simulink model "Arm11d"  (R2014b)
settings: Solver=ode23  StartTime=0.0  StopTime=4  MaxStep=0.005  RelTol=1e-3
values from neighbouring files (symbols this model uses):
  ArmIP = [2      0       -5;     -2      0       -5;           0      2       0;      0       -2      0;           -1     1       -6;     -1      -1      -6;           -1     1       -5;     -1      -1      -5;           0      -1.5    -6;      0      1.5     -15]    [params11c.m]    (also in params11cd.m; params11d.m)
  c = 1.12    [params11c.m]    (also in params11cd.m; params11d.m)
  d = 0.025    [params11c.m]    (also in params11cd.m; params11d.m)
  f1 = 0.82    [params11c.m]    (also in params11cd.m; params11d.m; piece5.m = sum(ar.*ar))
  f2 = 0.5    [params11c.m]    (also in params11cd.m; params11d.m; piece5.m = sum(cr.*cr))
  f3 = 0.43    [params11c.m]    (also in params11cd.m; params11d.m; piece5.m = sum(ar.*b))
  f4 = 0.58    [params11c.m]    (also in params11cd.m; params11d.m; piece5.m = sum(cr.*b))
  FarmIP = [0     1.5     -Larm-5;      0       -0.5    -Larm+3;            -1    1.5     -Larm-4]    [params11c.m]    (also in params11cd.m; params11d.m)
  Iarm = Iarm*10^(-4)    [params11c.m]    (also in params11cd.m; params11d.m)
  Ifarm = Ifarm*10^(-4)    [params11c.m]    (also in params11cd.m; params11d.m)
  kP = 2.58    [params11c.m]    (also in params11cd.m; params11d.m)
  Larm = 30    [params11c.m]    (also in params11cd.m; params11d.m)
  Lfarm = 26    [params11c.m]    (also in params11cd.m; params11d.m)
  Marm = dens*pi*(Rarm^2)*Larm    (= 2.35619449019)    [params11c.m]    (also in params11cd.m; params11d.m)
  Mfarm = dens*pi*(Rfarm^2)*Lfarm    (= 1.30690254389)    [params11c.m]    (also in params11cd.m; params11d.m)
  mu = 0.06    [params11c.m]    (also in params11cd.m; params11d.m)
  rhoP = 14.9    [params11c.m]    (also in params11cd.m; params11d.m)
  rlen = [13.8992; 12.5757; 9.1104; 7.1414; 17.4868; 17.7487; 18.8370;          17.8958; 33.5286; 22.2536; 16.9666]    [params11c.m]    (also in params11cd.m; params11d.m)
  tau = 0.01    [params11c.m]    (also in params11cd.m; params11d.m)
  tausq = tau^2    (= 0.0001)    [params11c.m]    (also in params11cd.m; params11d.m)
  vd = 0.15    [params11c.m]    (also in params11cd.m; params11d.m)
undefined symbols (not defined in the file or in its folder): geometry5, shaper2
libraries: mblibv1 x47, simulink x1
settings Model: Creator=sverduzco  LastModifiedBy=sergio
settings DataIOCC: SignalLoggingSaveFormat=ModelDataLogs
settings OptimizationCC: ExpressionDepthLimit=2147483647
settings DebuggingCC: UnderspecifiedInitializationDetection=Classic  MergeDetectMultiDrivingBlocksExec=none  FcnCallInpInsideContextMsg=UseLocalSettings  StateNameClashWarn=warning
settings GRTTargetCC: CombineOutputUpdateFcns=off  GRTInterface=on
settings SimMechanicsCC: VisOnUpdateDiagram=on  VisDuringSimulation=on

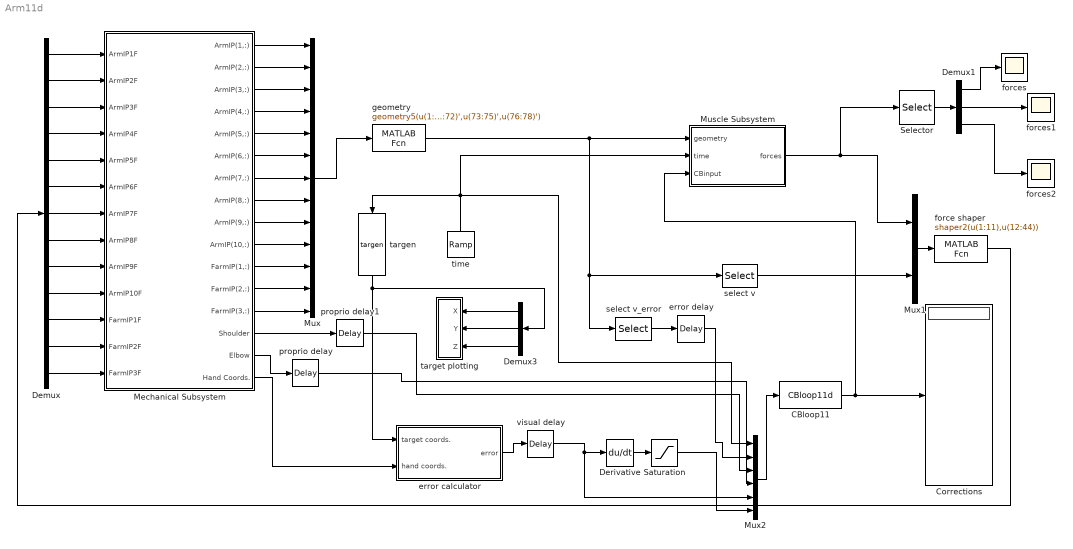
== system Arm11d ==
  CBloop11 : MATLABFcn  MATLABFcn=CBloop11d  OutputDimensions=11
  Corrections : Display
  Demux : Demux  Outputs=13
  Demux1 : Demux  Outputs=3
  Demux3 : Demux  Outputs=3
  Derivative : Derivative
  Mechanical Subsystem : Subsystem  Description=The arm insertion points are those of the ArmIP matrix in pointy.m, Ang2len2.m, and Quat2Euler.m, starting with CS3. The eight inputs are the force vectors applied at the eight points of ArmIP in the same order. The eight outputs are the coordinates of those insertion points.
  Muscle Subsystem : Subsystem
  Mux : Mux  Inputs=13
  Mux1 : Mux  Inputs=2
  Mux2 : Mux  Inputs=6
  Saturation : Saturate  UpperLimit=200  LowerLimit=0  ZeroCross=off
  Selector : Selector  InputPortWidth=11  Indices=[9 10 11]
  error calculator : Subsystem
  error delay : TransportDelay  DelayTime=d  BufferSize=30000  TransDelayFeedthrough=on  PadeOrder=1
  force shaper : MATLABFcn  MATLABFcn=shaper2(u(1:11),u(12:44))
  forces : Scope
      settings: TimeRange=6  YMin=0  YMax=30  SaveName=ScopeData3
  forces1 : Scope
      settings: TimeRange=6  YMin=0  YMax=30
  forces2 : Scope
      settings: TimeRange=6  YMin=0  YMax=30
  geometry : MATLABFcn  MATLABFcn=geometry5(u(1:3)',u(4:6)',u(7:9)',u(10:12)',u(13:15)',u(16:18)',u(19:21)',u(22:24)',u(25:27)',u(28:30)',u(31:33)',u(34:36)',u(37:39)',u(40:42)',u(43:45)',u(46:48)',u(49:51)',u(52:54)',u(55:57)',u(58:60)',u(61:63)',u(64:66)',u(67:69)',u(70:72)',u(73:75)',u(76:78)')
  proprio delay : TransportDelay  DelayTime=d  BufferSize=2000  TransDelayFeedthrough=on  PadeOrder=1
  proprio delay1 : TransportDelay  DelayTime=d  BufferSize=8000  TransDelayFeedthrough=on  PadeOrder=1
  select v : Selector  InputPortWidth=66  Indices=[34:66]
  select v_error : Selector  InputPortWidth=66  Indices=[1:11,23:33]
  targen : MATLABFcn  MATLABFcn=targen
  target plotting : Subsystem
  time : simulink/Sources/Ramp  slope=1  start=0  X0=0
  visual delay : TransportDelay  DelayTime=vd  BufferSize=8000  TransDelayFeedthrough=on  PadeOrder=1
  wires:
  Mux/1 -> geometry/1
  Mechanical Subsystem/1(ArmIP(1,:)) -> Mux/1
  Mechanical Subsystem/2(ArmIP(2,:)) -> Mux/2
  Mechanical Subsystem/3(ArmIP(3,:)) -> Mux/3
  Mechanical Subsystem/4(ArmIP(4,:)) -> Mux/4
  Mechanical Subsystem/5(ArmIP(5,:)) -> Mux/5
  Mechanical Subsystem/6(ArmIP(6,:)) -> Mux/6
  Mechanical Subsystem/7(ArmIP(7,:)) -> Mux/7
  Mechanical Subsystem/8(ArmIP(8,:)) -> Mux/8
  Mechanical Subsystem/9(ArmIP(9,:)) -> Mux/9
  Mechanical Subsystem/10(ArmIP(10,:)) -> Mux/10
  Mechanical Subsystem/11(FarmIP(1,:)) -> Mux/11
  Mechanical Subsystem/12(FarmIP(2,:)) -> Mux/12
  Mechanical Subsystem/13(FarmIP(3,:)) -> Mux/13
  Demux/1 -> Mechanical Subsystem/1(ArmIP1F)
  Demux/2 -> Mechanical Subsystem/2(ArmIP2F)
  Demux/3 -> Mechanical Subsystem/3(ArmIP3F)
  Demux/4 -> Mechanical Subsystem/4(ArmIP4F)
  Demux/5 -> Mechanical Subsystem/5(ArmIP5F)
  Demux/6 -> Mechanical Subsystem/6(ArmIP6F)
  Demux/7 -> Mechanical Subsystem/7(ArmIP7F)
  Demux/8 -> Mechanical Subsystem/8(ArmIP8F)
  Demux/9 -> Mechanical Subsystem/9(ArmIP9F)
  Demux/10 -> Mechanical Subsystem/10(ArmIP10F)
  Demux/11 -> Mechanical Subsystem/11(FarmIP1F)
  Demux/12 -> Mechanical Subsystem/12(FarmIP2F)
  Demux/13 -> Mechanical Subsystem/13(FarmIP3F)
  Muscle Subsystem/1(forces) -> Selector/1, Mux1/1
  select v/1 -> Mux1/2
  Mux1/1 -> force shaper/1
  geometry/1 -> select v/1, select v_error/1, Muscle Subsystem/1(geometry)
  force shaper/1 -> Demux/1
  time/1 -> Muscle Subsystem/2(time), targen/1, Mux2/1
  Demux3/3 -> target plotting/3(Z)
  Demux3/2 -> target plotting/2(Y)
  Demux3/1 -> target plotting/1(X)
  targen/1 -> Demux3/1, error calculator/1(target coords.)
  Mechanical Subsystem/16(Hand Coords.) -> error calculator/2(hand coords.)
  error calculator/1(error) -> visual delay/1
  Derivative/1 -> Saturation/1
  Mux2/1 -> CBloop11/1
  CBloop11/1 -> Muscle Subsystem/3(CBinput), Corrections/1
  Mechanical Subsystem/15(Elbow) -> proprio delay/1
  Mechanical Subsystem/14(Shoulder) -> proprio delay1/1
  select v_error/1 -> error delay/1
  Saturation/1 -> Mux2/6
  error delay/1 -> Mux2/2
  proprio delay/1 -> Mux2/4
  proprio delay1/1 -> Mux2/3
  visual delay/1 -> Derivative/1, Mux2/5
  Selector/1 -> Demux1/1
  Demux1/1 -> forces/1
  Demux1/2 -> forces1/1
  Demux1/3 -> forces2/1

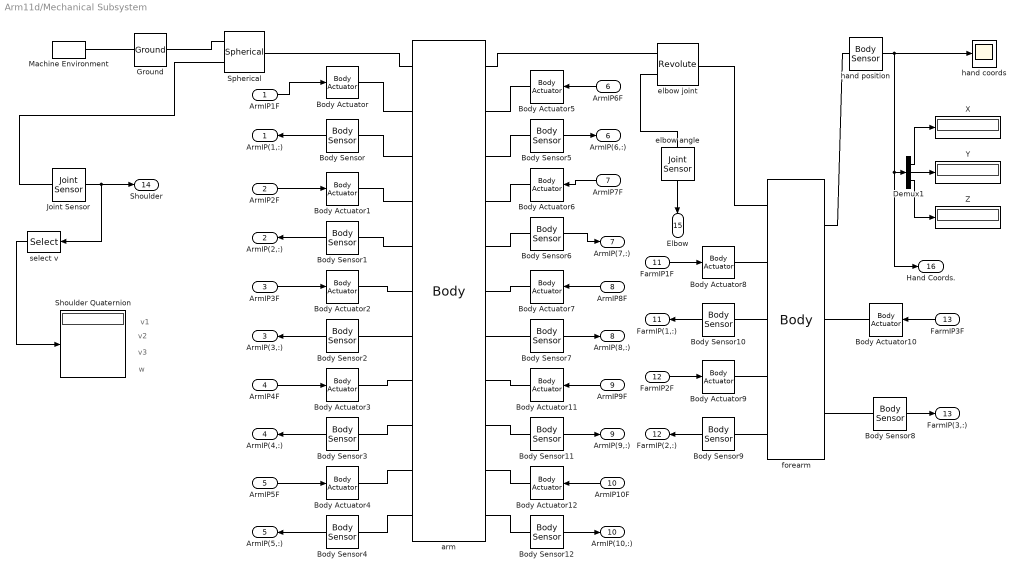
== system Arm11d/Mechanical Subsystem ==
  note: w
  note: v3
  note: v2
  note: v1
  ArmIP1F : Inport
  ArmIP2F : Inport  Port=2
  ArmIP3F : Inport  Port=3
  ArmIP4F : Inport  Port=4
  ArmIP5F : Inport  Port=5
  ArmIP6F : Inport  Port=6
  ArmIP7F : Inport  Port=7
  ArmIP8F : Inport  Port=8
  ArmIP9F : Inport  Port=9
  ArmIP10F : Inport  Port=10
  FarmIP1F : Inport  Port=11
  FarmIP2F : Inport  Port=12
  FarmIP3F : Inport  Port=13
  Body Actuator{,1..12} (13 alike) : mblibv1/Sensors &  Actuators/Body Actuator  UpdateFromCAD=off  PhysicalDomain=Mechanical  PortType=blob  ActuationStyle=Force  AngleUnits=deg  ArcVelocityUnits=deg/s  ArcAccelerationUnits=deg/s^2  CoordPositionUnits=m  VelocityUnits=m/s  AccelerationUnits=m/s^2  ForceUnits=N  TorqueUnits=N*m  ActiveIO=on  Width=3  DialogClass=MechanicalActuatorBlock  ReferenceFrame=Absolute (World)  Angle=off  CoordPosition=on  Force=on  Torque=off
  Body Sensor{,1..12} (13 alike) : mblibv1/Sensors &  Actuators/Body Sensor  UpdateFromCAD=off  PhysicalDomain=Mechanical  PortType=blob  Muxed=on  Pose=off  Angle=on  AngleUnits=deg  ArcVelocity=off  ArcVelocityUnits=deg/s  ArcAcceleration=off  ArcAccelerationUnits=deg/s^2  CoordPosition=on  CoordPositionUnits=cm  Velocity=on  VelocityUnits=cm/s  Acceleration=off  AccelerationUnits=m/s^2  Quaternion=on  QuaternionDT=off  QuaternionDDT=off  QuaternionUnits=off  OutputVector=[1]  ActiveIO=on  Width=6  DialogClass=MechanicalSensorBlock  ReferenceFrame=Absolute (World)
  Demux1 : Demux  Outputs=3
  Ground : mblibv1/Bodies/Ground  UpdateFromCAD=off  LeftPortType=env  RightPortType=workingframe  PhysicalDomain=Mechanical  DialogClass=GroundBlock  CoordPosition=[0 0 0]  CoordPositionUnits=cm  StateVectorMgrId=8  MachineId=[5 0]  ShowEnvPort=on  ParameterChecksum=[2283693424, 944707905, 1155320011, 4053348167]  TopologyChecksum=[2831574543, 1937149753, 2163190096, 3380941502]
  Joint Sensor : mblibv1/Sensors &  Actuators/Joint Sensor  UpdateFromCAD=off  PhysicalDomain=Mechanical  PortType=blob  Muxed=on  Pose=off  Angle=on  AngleUnits=deg  ArcVelocity=off  ArcVelocityUnits=deg/s  ArcAcceleration=off  ArcAccelerationUnits=deg/s^2  CoordPosition=on  CoordPositionUnits=m  Velocity=off  VelocityUnits=m/s  Acceleration=off  AccelerationUnits=m/s^2  Quaternion=on  QuaternionDT=on  QuaternionDDT=off  QuaternionUnits=off  OutputVector=[1]  ActiveIO=on  Width=8  DialogClass=MechanicalSensorBlock  Primitive=S  Force=off  ForceUnits=N  Torque=off  TorqueUnits=N*m  ReferenceFrame=Absolute (World)  ReactionSensedSide=Base  ReactionReferenceFrame=Absolute (World)  ReactionForce=off  ReactionForceUnits=N  ReactionMoment=off  ReactionMomentUnits=N*m
  Machine Environment : mblibv1/Bodies/Machine Environment  PortType=env  PhysicalDomain=Mechanical  DialogTemplateClass=MECH.MachineEnvironment  SyncWhenCopied=off  Gravity=[0 0 0]  GravityUnits=m/s^2  GravityAsSignal=off  Dimensionality=Auto-detect  AnalysisType=Forward dynamics  LinearAssemblyTolerance=1e-3  LinearAssemblyToleranceUnits=cm  AngularAssemblyTolerance=1e-3  AngularAssemblyToleranceUnits=rad  ConstraintSolverType=Stabilizing  ConstraintRelTolerance=1e-4  ConstraintAbsTolerance=1e-4  UseRobustSingularityHandling=off  RedundancyAnalysisToleranceType=Automatically select tolerance  RedundancyAnalysisTolerance=1e-14  StatePerturbationType=Fixed  PerturbationSize=1e-5  VisualizeMachine=on  BodyVisualizationType=Use model default body geometries  BodyColorSelMode=Use model default  DefaultBodyColor=[1 0 0]
  Shoulder Quaternion : Display
  Spherical : mblibv1/Joints/Spherical  LConnTagsString=__newl0|SA1  RConnTagsString=__newr0  UpdateFromCAD=off  NumSAPorts=1  CutJoint=off  MarkAsCut=off  Primitives=spherical  PrimitiveProps=S$World$[0 0 0]$spherical  DialogClass=JointBlock  SAxis=[0 0 0]
  X : Display
  Y : Display
  Z : Display
  arm : mblibv1/Bodies/Body  LConnTagsString=CS1|CS3|CS13|CS4|CS14|CS5|CS15|CS6|CS16|CS7|CS17  RConnTagsString=CS2|CS8|CS18|CS9|CS19|CS10|CS20|CS11|CS21|CS12|CS22  UpdateFromCAD=off  DialogClass=MechanicalBodyBlock  Mass=Marm  MassUnits=kg  InertiaUnits=kg*m^2  Inertia=Iarm  Shape=Cylinder  ShapeDims=[1 1]  ShapeUnits=m  ShapeUse=false  Density=1  DensityUnits=kg/m^3  DensityUse=false  GraphicsMode=MACHINE_DEFAULT  BodyColorSelMode=MACHINE_DEFAULT  BodyColor=[1 0 0]  AttachedToCS=CG  CG=Left$CG$[0 0 -(Larm/2)]$WORLD$WORLD$cm$[0 0 0]$Euler X-Y-Z$deg$WORLD$false$none  WorkingFrames=Left$CS1$[0 0 0]$World$World$cm$[0 0 0]$Euler X-Y-Z$deg$WORLD$true$none#Right$CS2$[0 0 -Larm]$World$World$cm$[0 0 0]$Euler X-Y-Z$deg$WORLD$true$none#Left$CS3$[ArmIP(1,1) ArmIP(1,2) ArmIP(1,3)]$World$World$cm$[0 0 0]$Euler X-Y-Z$deg$WORLD$true$none#Left$CS13$[ArmIP(1,1) ArmIP(1,2) ArmIP(1,3)]$World$World$cm$[0 0 0]$Euler X-Y-Z$deg$WORLD$true$none#Left$CS4$[ArmIP(2,1) ArmIP(2,2) ArmIP(2,3)]$World$World$cm$[0 0 0]$Euler X-Y-Z$deg$WORLD$true$none#Left$CS14$[ArmIP(2,1) ArmIP(2,2) ArmIP(2,3)]$World$World$cm$[0 0 0]$Euler X-Y-Z$deg$WORLD$true$none#Left$CS5$[ArmIP(3,1) ArmIP(3,2) ArmIP(3,3)]$World$World$cm$[0 0 0]$Euler X-Y-Z$deg$WORLD$true$none#Left$CS15$[ArmIP(3,1) ArmIP(3,2) ArmIP(3,3)]$World$World$cm$[0 0 0]$Euler X-Y-Z$deg$WORLD$true$none#Left$CS6$[ArmIP(4,1) ArmIP(4,2) ArmIP(4,3)]$World$World$cm$[0 0 0]$Euler X-Y-Z$deg$WORLD$true$none#Left$CS16$[ArmIP(4,1) ArmIP(4,2) ArmIP(4,3)]$World$World$cm$[0 0 0]$Euler X-Y-Z$deg$WORLD$true$none#Left$CS7$[ArmIP(5,1) ArmIP(5,2) ArmIP(5,3)]$World$World$cm$[0 0 0]$Euler X-Y-Z$deg$WORLD$true$none#Left$CS17$[ArmIP(5,1) ArmIP(5,2) ArmIP(5,3)]$World$World$cm$[0 0 0]$Euler X-Y-Z$deg$WORLD$true$none#Right$CS8$[ArmIP(6,1) ArmIP(6,2) ArmIP(6,3)]$World$World$cm$[0 0 0]$Euler X-Y-Z$deg$WORLD$true$none#Right$CS18$[ArmIP(6,1) ArmIP(6,2) ArmIP(6,3)]$World$World$cm$[0 0 0]$Euler X-Y-Z$deg$WORLD$true$none#Right$CS9$[ArmIP(7,1) ArmIP(7,2) ArmIP(7,3)]$World$World$cm$[0 0 0]$Euler X-Y-Z$deg$WORLD$true$none#Right$CS19$[ArmIP(7,1) ArmIP(7,2) ArmIP(7,3)]$World$World$cm$[0 0 0]$Euler X-Y-Z$deg$WORLD$true$none#Right$CS10$[ArmIP(8,1) ArmIP(8,2) ArmIP(8,3)]$World$World$cm$[0 0 0]$Euler X-Y-Z$deg$WORLD$true$none#Right$CS20$[ArmIP(8,1) ArmIP(8,2) ArmIP(8,3)]$World$World$cm$[0 0 0]$Euler X-Y-Z$deg$WORLD$true$none#Right$CS11$[ArmIP(9,1) ArmIP(9,2) ArmIP(9,3)]$World$World$cm$[0 0 0]$Euler X-Y-Z$deg$WORLD$true$none#Right$CS21$[ArmIP(9,1) ArmIP(9,2) ArmIP(9,3)]$World$World$cm$[0 0 0]$Euler X-Y-Z$deg$WORLD$true$none#Right$CS12$[ArmIP(10,1) ArmIP(10,2) ArmIP(10,3)]$World$World$cm$[0 0 0]$Euler X-Y-Z$deg$WORLD$true$none#Right$CS22$[ArmIP(10,1) ArmIP(10,2) ArmIP(10,3)]$World$World$cm$[0 0 0]$Euler X-Y-Z$deg$WORLD$true$none  CGPos=[0 0 -(Larm/2)]  CGRot=[0 0 0]  CS0Pos=[]  CS0Rot=[]  CS1Pos=[0 0 0]  CS1Rot=[0 0 0]  CS2Pos=[0 0 -Larm]  CS2Rot=[0 0 0]  CS3Pos=[ArmIP(1,1) ArmIP(1,2) ArmIP(1,3)]  CS3Rot=[0 0 0]  CS4Pos=[ArmIP(2,1) ArmIP(2,2) ArmIP(2,3)]  CS4Rot=[0 0 0]  CS5Pos=[ArmIP(3,1) ArmIP(3,2) ArmIP(3,3)]  CS5Rot=[0 0 0]  CS6Pos=[ArmIP(4,1) ArmIP(4,2) ArmIP(4,3)]  CS6Rot=[0 0 0]  CS7Pos=[ArmIP(5,1) ArmIP(5,2) ArmIP(5,3)]  CS7Rot=[0 0 0]  CS8Pos=[ArmIP(6,1) ArmIP(6,2) ArmIP(6,3)]  CS8Rot=[0 0 0]  CS9Pos=[ArmIP(7,1) ArmIP(7,2) ArmIP(7,3)]  CS9Rot=[0 0 0]  CS10Pos=[ArmIP(8,1) ArmIP(8,2) ArmIP(8,3)]  CS10Rot=[0 0 0]  CS11Pos=[ArmIP(9,1) ArmIP(9,2) ArmIP(9,3)]  CS11Rot=[0 0 0]  CS12Pos=[ArmIP(10,1) ArmIP(10,2) ArmIP(10,3)]  CS12Rot=[0 0 0]  CS13Pos=[ArmIP(1,1) ArmIP(1,2) ArmIP(1,3)]  CS13Rot=[0 0 0]  CS14Pos=[ArmIP(2,1) ArmIP(2,2) ArmIP(2,3)]  CS14Rot=[0 0 0]  CS15Pos=[ArmIP(3,1) ArmIP(3,2) ArmIP(3,3)]  CS15Rot=[0 0 0]  CS16Pos=[ArmIP(4,1) ArmIP(4,2) ArmIP(4,3)]  CS16Rot=[0 0 0]  CS17Pos=[ArmIP(5,1) ArmIP(5,2) ArmIP(5,3)]  CS17Rot=[0 0 0]  CS18Pos=[ArmIP(6,1) ArmIP(6,2) ArmIP(6,3)]  CS18Rot=[0 0 0]  CS19Pos=[ArmIP(7,1) ArmIP(7,2) ArmIP(7,3)]  CS19Rot=[0 0 0]  CS20Pos=[ArmIP(8,1) ArmIP(8,2) ArmIP(8,3)]  CS20Rot=[0 0 0]
  elbow angle : mblibv1/Sensors &  Actuators/Joint Sensor  UpdateFromCAD=off  PhysicalDomain=Mechanical  PortType=blob  Muxed=on  Pose=off  Angle=on  AngleUnits=rad  ArcVelocity=on  ArcVelocityUnits=rad/s  ArcAcceleration=off  ArcAccelerationUnits=deg/s^2  CoordPosition=on  CoordPositionUnits=m  Velocity=off  VelocityUnits=m/s  Acceleration=off  AccelerationUnits=m/s^2  Quaternion=on  QuaternionDT=off  QuaternionDDT=off  QuaternionUnits=off  OutputVector=[1]  ActiveIO=on  Width=2  DialogClass=MechanicalSensorBlock  Primitive=R1  Force=off  ForceUnits=N  Torque=off  TorqueUnits=N*m  ReferenceFrame=Absolute (World)  ReactionSensedSide=Base  ReactionReferenceFrame=Local (Body CS)  ReactionForce=off  ReactionForceUnits=N  ReactionMoment=off  ReactionMomentUnits=N*m
  elbow joint : mblibv1/Joints/Revolute  LConnTagsString=__newl0|SA1  RConnTagsString=__newr0  UpdateFromCAD=off  NumSAPorts=1  CutJoint=off  MarkAsCut=off  Primitives=prismatic  PrimitiveProps=R1$Base$[1 0 0]$revolute  DialogClass=JointBlock  R1Axis=[1 0 0]
  forearm : mblibv1/Bodies/Body  LConnTagsString=CS1|CS3|CS6|CS4|CS7  RConnTagsString=CS2|CS5|CS8  UpdateFromCAD=off  DialogClass=MechanicalBodyBlock  Mass=Mfarm  MassUnits=kg  InertiaUnits=kg*m^2  Inertia=Ifarm  Shape=Cylinder  ShapeDims=[1 1]  ShapeUnits=m  ShapeUse=false  Density=1  DensityUnits=kg/m^3  DensityUse=false  GraphicsMode=MACHINE_DEFAULT  BodyColorSelMode=MACHINE_DEFAULT  BodyColor=[1 0 0]  AttachedToCS=CG  CG=Left$CG$[0 0 -(Larm+(Lfarm/2))]$WORLD$WORLD$cm$[0 0 0]$Euler X-Y-Z$deg$WORLD$false$none  WorkingFrames=Left$CS1$[0 0 -Larm]$World$World$cm$[0 0 0]$Euler X-Y-Z$deg$WORLD$true$none#Right$CS2$[0 0 -(Larm+Lfarm)]$World$World$cm$[0 0 0]$Euler X-Y-Z$deg$WORLD$true$none#Left$CS3$[FarmIP(1,1) FarmIP(1,2) FarmIP(1,3)]$World$World$cm$[0 0 0]$Euler X-Y-Z$deg$WORLD$true$none#Left$CS6$[FarmIP(1,1) FarmIP(1,2) FarmIP(1,3)]$World$World$cm$[0 0 0]$Euler X-Y-Z$deg$WORLD$true$none#Left$CS4$[FarmIP(2,1) FarmIP(2,2) FarmIP(2,3)]$World$World$cm$[0 0 0]$Euler X-Y-Z$deg$WORLD$true$none#Left$CS7$[FarmIP(2,1) FarmIP(2,2) FarmIP(2,3)]$World$World$cm$[0 0 0]$Euler X-Y-Z$deg$WORLD$true$none#Right$CS5$[FarmIP(3,1) FarmIP(3,2) FarmIP(3,3)]$World$World$cm$[0 0 0]$Euler X-Y-Z$deg$WORLD$true$none#Right$CS8$[FarmIP(3,1) FarmIP(3,2) FarmIP(3,3)]$World$World$cm$[0 0 0]$Euler X-Y-Z$deg$WORLD$true$none  CGPos=[0 0 -(Larm+(Lfarm/2))]  CGRot=[0 0 0]  CS0Pos=[]  CS0Rot=[]  CS1Pos=[0 0 -Larm]  CS1Rot=[0 0 0]  CS2Pos=[0 0 -(Larm+Lfarm)]  CS2Rot=[0 0 0]  CS3Pos=[FarmIP(1,1) FarmIP(1,2) FarmIP(1,3)]  CS3Rot=[0 0 0]  CS4Pos=[FarmIP(2,1) FarmIP(2,2) FarmIP(2,3)]  CS4Rot=[0 0 0]  CS5Pos=[FarmIP(3,1) FarmIP(3,2) FarmIP(3,3)]  CS5Rot=[0 0 0]  CS6Pos=[FarmIP(1,1) FarmIP(1,2) FarmIP(1,3)]  CS6Rot=[0 0 0]  CS7Pos=[FarmIP(2,1) FarmIP(2,2) FarmIP(2,3)]  CS7Rot=[0 0 0]  CS8Pos=[FarmIP(3,1) FarmIP(3,2) FarmIP(3,3)]  CS8Rot=[0 0 0]  CS9Pos=[]  CS9Rot=[]  CS10Pos=[]  CS10Rot=[]  CS11Pos=[]  CS11Rot=[]  CS12Pos=[]  CS12Rot=[]  CS13Pos=[]  CS13Rot=[]  CS14Pos=[]  CS14Rot=[]  CS15Pos=[]  CS15Rot=[]  CS16Pos=[]  CS16Rot=[]  CS17Pos=[]  CS17Rot=[]  CS18Pos=[]  CS18Rot=[]  CS19Pos=[]  CS19Rot=[]  CS20Pos=[]  CS20Rot=[]
  hand coords : Scope
      settings: SaveName=ScopeData2
  hand position : mblibv1/Sensors &  Actuators/Body Sensor  UpdateFromCAD=off  PhysicalDomain=Mechanical  PortType=blob  Muxed=on  Pose=off  Angle=on  AngleUnits=deg  ArcVelocity=off  ArcVelocityUnits=deg/s  ArcAcceleration=off  ArcAccelerationUnits=deg/s^2  CoordPosition=on  CoordPositionUnits=cm  Velocity=off  VelocityUnits=m/s  Acceleration=off  AccelerationUnits=m/s^2  Quaternion=on  QuaternionDT=off  QuaternionDDT=off  QuaternionUnits=off  OutputVector=[1]  ActiveIO=on  Width=3  DialogClass=MechanicalSensorBlock  ReferenceFrame=Absolute (World)
  select v : Selector  InputPortWidth=8  Indices=[1:4]
  ArmIP(1,:) : Outport
  ArmIP(2,:) : Outport  Port=2
  ArmIP(3,:) : Outport  Port=3
  ArmIP(4,:) : Outport  Port=4
  ArmIP(5,:) : Outport  Port=5
  ArmIP(6,:) : Outport  Port=6
  ArmIP(7,:) : Outport  Port=7
  ArmIP(8,:) : Outport  Port=8
  ArmIP(9,:) : Outport  Port=9
  ArmIP(10,:) : Outport  Port=10
  FarmIP(1,:) : Outport  Port=11
  FarmIP(2,:) : Outport  Port=12
  FarmIP(3,:) : Outport  Port=13
  Shoulder : Outport  Port=14
  Elbow : Outport  Port=15
  Hand Coords. : Outport  Port=16
  wires:
  Joint Sensor/1 -> Shoulder/1, select v/1
  hand position/1 -> hand coords/1, Demux1/1, Hand Coords./1
  Demux1/1 -> X/1
  Demux1/2 -> Y/1
  Demux1/3 -> Z/1
  ArmIP1F/1 -> Body Actuator/1
  ArmIP2F/1 -> Body Actuator1/1
  ArmIP3F/1 -> Body Actuator2/1
  ArmIP4F/1 -> Body Actuator3/1
  ArmIP5F/1 -> Body Actuator4/1
  ArmIP6F/1 -> Body Actuator5/1
  ArmIP7F/1 -> Body Actuator6/1
  ArmIP8F/1 -> Body Actuator7/1
  Body Sensor/1 -> ArmIP(1,:)/1
  Body Sensor1/1 -> ArmIP(2,:)/1
  Body Sensor2/1 -> ArmIP(3,:)/1
  Body Sensor3/1 -> ArmIP(4,:)/1
  Body Sensor4/1 -> ArmIP(5,:)/1
  Body Sensor5/1 -> ArmIP(6,:)/1
  Body Sensor6/1 -> ArmIP(7,:)/1
  Body Sensor7/1 -> ArmIP(8,:)/1
  FarmIP3F/1 -> Body Actuator10/1
  FarmIP1F/1 -> Body Actuator8/1
  FarmIP2F/1 -> Body Actuator9/1
  Body Sensor9/1 -> FarmIP(2,:)/1
  Body Sensor10/1 -> FarmIP(1,:)/1
  Body Sensor8/1 -> FarmIP(3,:)/1
  ArmIP9F/1 -> Body Actuator11/1
  ArmIP10F/1 -> Body Actuator12/1
  Body Sensor11/1 -> ArmIP(9,:)/1
  Body Sensor12/1 -> ArmIP(10,:)/1
  elbow angle/1 -> Elbow/1
  select v/1 -> Shoulder Quaternion/1
  connections:
  Machine Environment/RConn1 -- Ground/LConn1
  Ground/RConn1 -- Spherical/LConn1
  Spherical/LConn2 -- Joint Sensor/LConn1
  Spherical/RConn1 -- arm/LConn1
  arm/RConn1 -- elbow joint/LConn1
  elbow joint/RConn1 -- forearm/LConn1
  forearm/RConn1 -- hand position/LConn1
  elbow joint/LConn2 -- elbow angle/LConn1
  Body Actuator8/RConn1 -- forearm/LConn2
  Body Sensor10/LConn1 -- forearm/LConn3
  Body Actuator9/RConn1 -- forearm/LConn4
  Body Sensor9/LConn1 -- forearm/LConn5
  forearm/RConn3 -- Body Sensor8/LConn1
  forearm/RConn2 -- Body Actuator10/RConn1
  Body Actuator/RConn1 -- arm/LConn2
  Body Sensor/LConn1 -- arm/LConn3
  Body Actuator1/RConn1 -- arm/LConn4
  Body Sensor1/LConn1 -- arm/LConn5
  arm/LConn6 -- Body Actuator2/RConn1
  arm/LConn7 -- Body Sensor2/LConn1
  arm/LConn8 -- Body Actuator3/RConn1
  arm/LConn9 -- Body Sensor3/LConn1
  arm/LConn10 -- Body Actuator4/RConn1
  arm/LConn11 -- Body Sensor4/LConn1
  Body Actuator5/RConn1 -- arm/RConn2
  Body Sensor5/LConn1 -- arm/RConn3
  Body Actuator6/RConn1 -- arm/RConn4
  Body Sensor6/LConn1 -- arm/RConn5
  Body Actuator7/RConn1 -- arm/RConn6
  Body Sensor7/LConn1 -- arm/RConn7
  Body Actuator11/RConn1 -- arm/RConn8
  Body Sensor11/LConn1 -- arm/RConn9
  Body Actuator12/RConn1 -- arm/RConn10
  Body Sensor12/LConn1 -- arm/RConn11

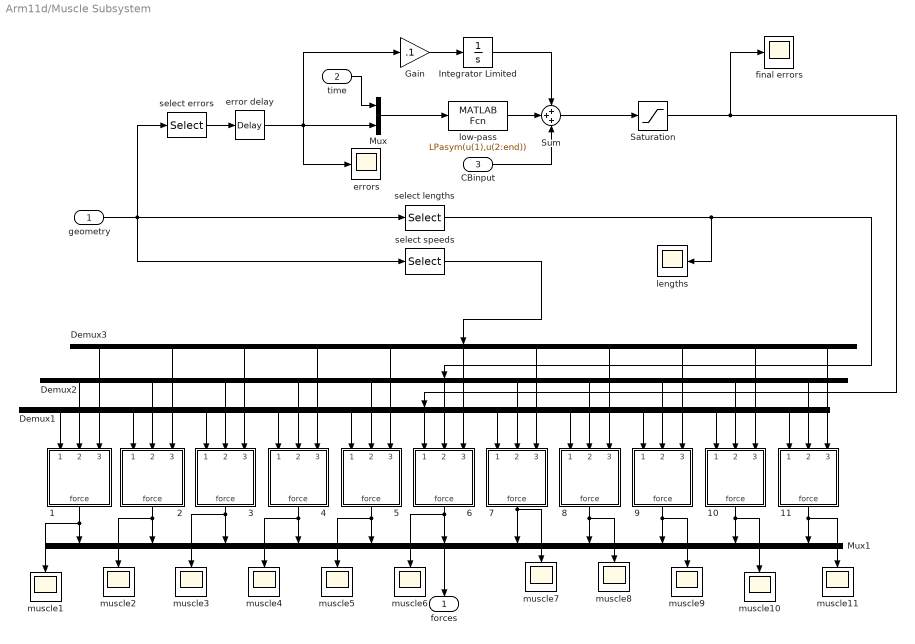
== system Arm11d/Muscle Subsystem ==
  geometry : Inport
  time : Inport  Port=2
  CBinput : Inport  Port=3
  1 : Subsystem
  10 : Subsystem
  11 : Subsystem
  2 : Subsystem
  3 : Subsystem
  4 : Subsystem
  5 : Subsystem
  6 : Subsystem
  7 : Subsystem
  8 : Subsystem
  9 : Subsystem
  Demux1 : Demux  Outputs=11
  Demux2 : Demux  Outputs=11
  Demux3 : Demux  Outputs=11
  Gain : Gain  Gain=.1
  Integrator Limited : Integrator  LimitOutput=on  UpperSaturationLimit=1  LowerSaturationLimit=-.1
  Mux : Mux  Inputs=2
  Mux1 : Mux  Inputs=11
  Saturation : Saturate  UpperLimit=8  LowerLimit=0
  Sum : Sum  Inputs=+++
  error delay : TransportDelay  DelayTime=d  BufferSize=20000  TransDelayFeedthrough=on  PadeOrder=1
  errors : Scope
      settings: TimeRange=6  YMin=-1.75  YMax=1  SaveName=ScopeData5
  final errors : Scope
      settings: TimeRange=6  YMin=0  YMax=0.5  SaveName=ScopeData4
  lengths : Scope
      settings: TimeRange=6  YMin=5  YMax=37.5  SaveName=ScopeData9
  low-pass : MATLABFcn  MATLABFcn=LPasym(u(1),u(2:end))
  muscle{1..11} (11 alike) : Scope
      muscle1 settings: TimeRange=6  YMin=0  YMax=17.5  SaveName=ScopeData12
      muscle10 settings: TimeRange=6  YMin=0  YMax=20  SaveName=ScopeData8
      muscle11 settings: TimeRange=6  YMin=0  YMax=8  SaveName=ScopeData10
      muscle2 settings: TimeRange=6  YMin=-1  YMax=1  SaveName=ScopeData6
      muscle3 settings: TimeRange=6  YMin=0.25  YMax=0.55  SaveName=ScopeData13
      muscle4 settings: TimeRange=6  YMin=0  YMax=100  SaveName=ScopeData14
      muscle5 settings: TimeRange=6  YMin=0  YMax=50  SaveName=ScopeData15
      muscle6 settings: TimeRange=6  YMin=0  YMax=6  SaveName=ScopeData16
      muscle7 settings: TimeRange=6  YMin=0  YMax=15  SaveName=ScopeData17
      muscle8 settings: TimeRange=6  YMin=0  YMax=6  SaveName=ScopeData7
      muscle9 settings: TimeRange=6  YMin=0  YMax=7  SaveName=ScopeData11
  select errors : Selector  InputPortWidth=66  Indices=[23:33]
  select lengths : Selector  InputPortWidth=66  Indices=[1:11]
  select speeds : Selector  InputPortWidth=66  Indices=[12:22]
  forces : Outport
  wires:
  Demux1/1 -> 1/1(error)
  Demux2/1 -> 1/2(length)
  Demux3/1 -> 1/3(speed)
  Demux1/2 -> 2/1(error)
  Demux2/2 -> 2/2(length)
  Demux3/2 -> 2/3(speed)
  Demux1/3 -> 3/1(error)
  Demux2/3 -> 3/2(length)
  Demux3/3 -> 3/3(speed)
  Demux1/4 -> 4/1(error)
  Demux2/4 -> 4/2(length)
  Demux3/4 -> 4/3(speed)
  Demux1/5 -> 5/1(error)
  Demux2/5 -> 5/2(length)
  Demux3/5 -> 5/3(speed)
  Demux1/6 -> 6/1(error)
  Demux2/6 -> 6/2(length)
  Demux3/6 -> 6/3(speed)
  Demux1/7 -> 7/1(error)
  Demux2/7 -> 7/2(length)
  Demux3/7 -> 7/3(speed)
  Demux1/8 -> 8/1(error)
  Demux2/8 -> 8/2(length)
  Demux3/8 -> 8/3(speed)
  Demux1/9 -> 9/1(error)
  Demux2/9 -> 9/2(length)
  Demux3/9 -> 9/3(speed)
  Demux1/10 -> 10/1(error)
  Demux2/10 -> 10/2(length)
  Demux3/10 -> 10/3(speed)
  select lengths/1 -> lengths/1, Demux2/1
  select speeds/1 -> Demux3/1
  1/1(force) -> Mux1/1, muscle1/1
  2/1(force) -> Mux1/2, muscle2/1
  3/1(force) -> Mux1/3, muscle3/1
  4/1(force) -> Mux1/4, muscle4/1
  5/1(force) -> Mux1/5, muscle5/1
  6/1(force) -> Mux1/6, muscle6/1
  7/1(force) -> Mux1/7, muscle7/1
  8/1(force) -> Mux1/8, muscle8/1
  9/1(force) -> Mux1/9, muscle9/1
  10/1(force) -> Mux1/10, muscle10/1
  geometry/1 -> select speeds/1, select lengths/1, select errors/1
  Mux1/1 -> forces/1
  11/1(force) -> Mux1/11, muscle11/1
  Demux1/11 -> 11/1(error)
  Demux2/11 -> 11/2(length)
  Demux3/11 -> 11/3(speed)
  time/1 -> Mux/1
  select errors/1 -> error delay/1
  Mux/1 -> low-pass/1
  low-pass/1 -> Sum/2
  Integrator Limited/1 -> Sum/1
  Gain/1 -> Integrator Limited/1
  Saturation/1 -> Demux1/1, final errors/1
  CBinput/1 -> Sum/3
  Sum/1 -> Saturation/1
  error delay/1 -> errors/1, Mux/2, Gain/1

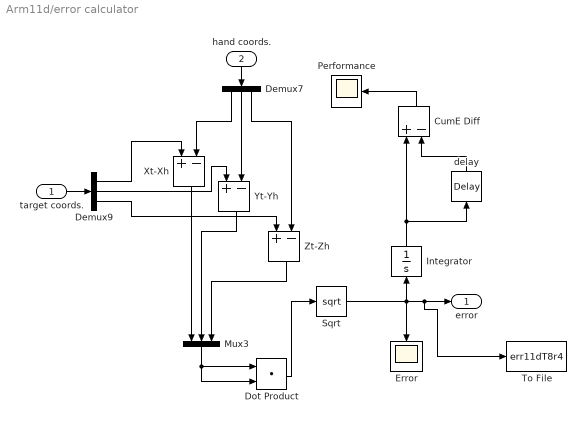
== system Arm11d/error calculator ==
  target coords. : Inport
  hand coords. : Inport  Port=2
  CumE Diff : Sum  Inputs=+-
  Demux7 : Demux  Outputs=3
  Demux9 : Demux  Outputs=3
  Dot Product : DotProduct  InputSameDT=on  OutDataTypeStr=Inherit: Inherit via internal rule
  Error : Scope
      settings: TimeRange=5  YMin=0  YMax=50  SaveName=ScopeData13
  Integrator : Integrator
  Mux3 : Mux  Inputs=3
  Performance : Scope
      settings: TimeRange=16  YMin=0  YMax=100  SaveName=ScopeData17
  Sqrt : Sqrt  SaturateOnIntegerOverflow=on
  To File : ToFile  Filename=err11dT8r4  MatrixName=err11dT8r4  SaveFormat=Timeseries
  Xt-Xh : Sum  Inputs=+-
  Yt-Yh : Sum  Inputs=+-
  Zt-Zh : Sum  Inputs=+-
  delay : TransportDelay  DelayTime=10  BufferSize=4800
  error : Outport
  wires:
  Demux7/1 -> Xt-Xh/2
  Integrator/1 -> delay/1, CumE Diff/1
  Demux9/1 -> Xt-Xh/1
  Demux9/2 -> Yt-Yh/1
  hand coords./1 -> Demux7/1
  target coords./1 -> Demux9/1
  Dot Product/1 -> Sqrt/1
  Sqrt/1 -> Error/1, Integrator/1, To File/1, error/1
  CumE Diff/1 -> Performance/1
  delay/1 -> CumE Diff/2
  Demux9/3 -> Zt-Zh/1
  Demux7/3 -> Zt-Zh/2
  Xt-Xh/1 -> Mux3/1
  Demux7/2 -> Yt-Yh/2
  Yt-Yh/1 -> Mux3/2
  Zt-Zh/1 -> Mux3/3
  Mux3/1 -> Dot Product/1, Dot Product/2

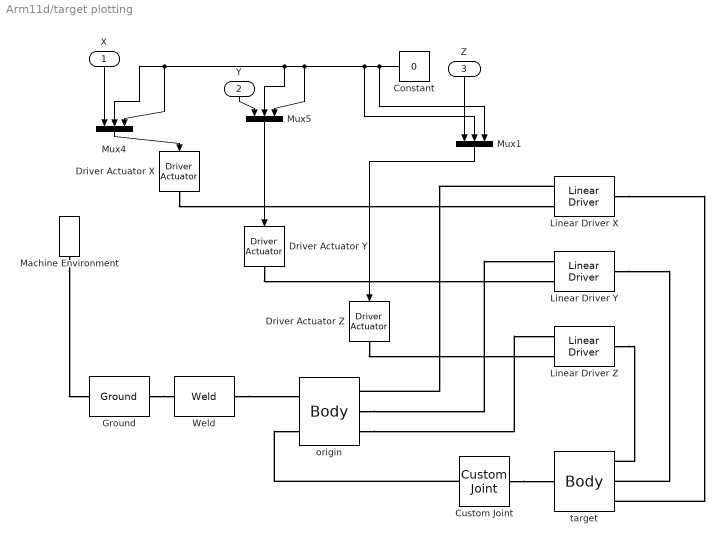
== system Arm11d/target plotting ==
  X : Inport
  Y : Inport  Port=2
  Z : Inport  Port=3
  Constant : Constant  Value=0
  Custom Joint : mblibv1/Joints/Custom Joint  LConnTagsString=__newl0  RConnTagsString=__newr0  UpdateFromCAD=off  NumSAPorts=0  CutJoint=off  MarkAsCut=off  Primitives=prismatic  PrimitiveProps=P1$World$[1 0 0]$Prismatic#P2$World$[0 1 0]$Prismatic#P3$World$[0 0 1]$Prismatic  DialogClass=JointBlock  R1Axis=[]  R2Axis=[]  R3Axis=[]  P1Axis=[1 0 0]  P2Axis=[0 1 0]  P3Axis=[0 0 1]  SAxis=[]
  Driver Actuator X : mblibv1/Sensors &  Actuators/Driver Actuator  UpdateFromCAD=off  PhysicalDomain=Mechanical  DialogClass=ConstraintActuatorBlock  PortType=blob  AngleUnits=deg  ArcVelocityUnits=deg/s  ArcAccelerationUnits=deg/s^2  CoordPositionUnits=cm  VelocityUnits=cm/s  AccelerationUnits=cm/s^2  ActiveIO=on  Width=3
  Driver Actuator Y : mblibv1/Sensors &  Actuators/Driver Actuator  UpdateFromCAD=off  PhysicalDomain=Mechanical  DialogClass=ConstraintActuatorBlock  PortType=blob  AngleUnits=deg  ArcVelocityUnits=deg/s  ArcAccelerationUnits=deg/s^2  CoordPositionUnits=cm  VelocityUnits=cm/s  AccelerationUnits=cm/s^2  ActiveIO=on  Width=3
  Driver Actuator Z : mblibv1/Sensors &  Actuators/Driver Actuator  UpdateFromCAD=off  PhysicalDomain=Mechanical  DialogClass=ConstraintActuatorBlock  PortType=blob  AngleUnits=deg  ArcVelocityUnits=deg/s  ArcAccelerationUnits=deg/s^2  CoordPositionUnits=cm  VelocityUnits=cm/s  AccelerationUnits=cm/s^2  ActiveIO=on  Width=3
  Ground : mblibv1/Bodies/Ground  UpdateFromCAD=off  LeftPortType=env  RightPortType=workingframe  PhysicalDomain=Mechanical  DialogClass=GroundBlock  CoordPosition=[0 0 0]  CoordPositionUnits=cm  StateVectorMgrId=9  MachineId=[5 1]  ShowEnvPort=on  ParameterChecksum=[3808905041, 2576024276, 3612694341, 1264581059]  TopologyChecksum=[2403528271, 2533162851, 2656289086, 1853666437]
  Linear Driver X : mblibv1/Constraints &  Drivers/Linear Driver  LConnTagsString=__newl0|SA1  RConnTagsString=__newr0  UpdateFromCAD=off  DialogClass=LinearDriverConstraint  NumSAPorts=1  GlobalCoordinate=X
  Linear Driver Y : mblibv1/Constraints &  Drivers/Linear Driver  LConnTagsString=__newl0|SA1  RConnTagsString=__newr0  UpdateFromCAD=off  DialogClass=LinearDriverConstraint  NumSAPorts=1  GlobalCoordinate=Y
  Linear Driver Z : mblibv1/Constraints &  Drivers/Linear Driver  LConnTagsString=__newl0|SA1  RConnTagsString=__newr0  UpdateFromCAD=off  DialogClass=LinearDriverConstraint  NumSAPorts=1  GlobalCoordinate=Z
  Machine Environment : mblibv1/Bodies/Machine Environment  PortType=env  PhysicalDomain=Mechanical  DialogTemplateClass=MECH.MachineEnvironment  SyncWhenCopied=off  Gravity=[0 0 0]  GravityUnits=m/s^2  GravityAsSignal=off  Dimensionality=Auto-detect  AnalysisType=Forward dynamics  LinearAssemblyTolerance=1e-3  LinearAssemblyToleranceUnits=cm  AngularAssemblyTolerance=1e-3  AngularAssemblyToleranceUnits=rad  ConstraintSolverType=Tolerancing  ConstraintRelTolerance=1e-4  ConstraintAbsTolerance=1e-4  UseRobustSingularityHandling=off  RedundancyAnalysisToleranceType=Automatically select tolerance  RedundancyAnalysisTolerance=1e-14  StatePerturbationType=Fixed  PerturbationSize=1e-5  VisualizeMachine=on  BodyVisualizationType=Equivalent ellipsoid from mass properties  BodyColorSelMode=Use model default  DefaultBodyColor=[1 0 0]
  Mux1 : Mux  Inputs=3
  Mux4 : Mux  Inputs=3
  Mux5 : Mux  Inputs=3
  Weld : mblibv1/Joints/Weld  LConnTagsString=__newl0  RConnTagsString=__newr0  UpdateFromCAD=off  NumSAPorts=0  CutJoint=off  MarkAsCut=off  Primitives=weld  PrimitiveProps=W$World$[0 0 0]$weld  DialogClass=JointBlock  WAxis=[0 0 0]
  origin : mblibv1/Bodies/Body  LConnTagsString=CS1|CS2  RConnTagsString=CS3|CS4|CS5  UpdateFromCAD=off  DialogClass=MechanicalBodyBlock  Mass=1  MassUnits=kg  InertiaUnits=kg*m^2  Inertia=(1e-5)*eye(3)  Shape=Cylinder  ShapeDims=[1 1]  ShapeUnits=m  ShapeUse=false  Density=1  DensityUnits=kg/m^3  DensityUse=false  GraphicsMode=MACHINE_DEFAULT  BodyColorSelMode=MACHINE_DEFAULT  BodyColor=[1 0 0]  AttachedToCS=CG  CG=Left$CG$[0 0 0]$WORLD$WORLD$cm$[0 0 0]$Euler X-Y-Z$deg$WORLD$false$none  WorkingFrames=Right$CS3$[0 0 0]$WORLD$WORLD$cm$[0 0 0]$Euler X-Y-Z$deg$WORLD$true$none#Right$CS4$[0 0 0]$WORLD$WORLD$cm$[0 0 0]$Euler X-Y-Z$deg$WORLD$true$none#Right$CS5$[0 0 0]$WORLD$WORLD$cm$[0 0 0]$Euler X-Y-Z$deg$WORLD$true$none#Left$CS1$[0 0 0]$CG$CG$cm$[0 0 0]$Euler X-Y-Z$deg$WORLD$true$none#Left$CS2$[0 0 0]$World$World$cm$[0 0 0]$Euler X-Y-Z$deg$WORLD$true$none  CGPos=[0 0 0]  CGRot=[0 0 0]  CS0Pos=[]  CS0Rot=[]  CS1Pos=[0 0 0]  CS1Rot=[0 0 0]  CS2Pos=[0 0 0]  CS2Rot=[0 0 0]  CS3Pos=[0 0 0]  CS3Rot=[0 0 0]  CS4Pos=[0 0 0]  CS4Rot=[0 0 0]  CS5Pos=[0 0 0]  CS5Rot=[0 0 0]  CS6Pos=[]  CS6Rot=[]  CS7Pos=[]  CS7Rot=[]  CS8Pos=[]  CS8Rot=[]  CS9Pos=[]  CS9Rot=[]  CS10Pos=[]  CS10Rot=[]  CS11Pos=[]  CS11Rot=[]  CS12Pos=[]  CS12Rot=[]  CS13Pos=[]  CS13Rot=[]  CS14Pos=[]  CS14Rot=[]  CS15Pos=[]  CS15Rot=[]  CS16Pos=[]  CS16Rot=[]  CS17Pos=[]  CS17Rot=[]  CS18Pos=[]  CS18Rot=[]  CS19Pos=[]  CS19Rot=[]  CS20Pos=[]  CS20Rot=[]
  target : mblibv1/Bodies/Body  LConnTagsString=CS1  RConnTagsString=CS4|CS3|CS2  UpdateFromCAD=off  DialogClass=MechanicalBodyBlock  Mass=.1  MassUnits=kg  InertiaUnits=kg*m^2  Inertia=(1e-5)*eye(3)  Shape=Cylinder  ShapeDims=[1 1]  ShapeUnits=m  ShapeUse=false  Density=1  DensityUnits=kg/m^3  DensityUse=false  GraphicsMode=MACHINE_DEFAULT  BodyColorSelMode=COLORPALETTE  BodyColor=[0 1 0]  AttachedToCS=CG  CG=Left$CG$[0 0 0]$WORLD$WORLD$cm$[0 0 0]$Euler X-Y-Z$deg$WORLD$false$none  WorkingFrames=Right$CS4$[0 0 0]$WORLD$WORLD$cm$[0 0 0]$Euler X-Y-Z$deg$WORLD$true$none#Right$CS3$[0 0 0]$WORLD$WORLD$cm$[0 0 0]$Euler X-Y-Z$deg$WORLD$true$none#Left$CS1$[0 0 0]$CG$CG$cm$[0 0 0]$Euler X-Y-Z$deg$WORLD$true$none#Right$CS2$[0 0 0]$World$World$cm$[0 0 0]$Euler X-Y-Z$deg$WORLD$true$none  CGPos=[0 0 0]  CGRot=[0 0 0]  CS0Pos=[]  CS0Rot=[]  CS1Pos=[0 0 0]  CS1Rot=[0 0 0]  CS2Pos=[0 0 0]  CS2Rot=[0 0 0]  CS3Pos=[0 0 0]  CS3Rot=[0 0 0]  CS4Pos=[0 0 0]  CS4Rot=[0 0 0]  CS5Pos=[]  CS5Rot=[]  CS6Pos=[]  CS6Rot=[]  CS7Pos=[]  CS7Rot=[]  CS8Pos=[]  CS8Rot=[]  CS9Pos=[]  CS9Rot=[]  CS10Pos=[]  CS10Rot=[]  CS11Pos=[]  CS11Rot=[]  CS12Pos=[]  CS12Rot=[]  CS13Pos=[]  CS13Rot=[]  CS14Pos=[]  CS14Rot=[]  CS15Pos=[]  CS15Rot=[]  CS16Pos=[]  CS16Rot=[]  CS17Pos=[]  CS17Rot=[]  CS18Pos=[]  CS18Rot=[]  CS19Pos=[]  CS19Rot=[]  CS20Pos=[]  CS20Rot=[]
  wires:
  Mux4/1 -> Driver Actuator X/1
  Constant/1 -> Mux5/3, Mux4/2, Mux4/3, Mux5/2, Mux1/2, Mux1/3
  Mux5/1 -> Driver Actuator Y/1
  X/1 -> Mux4/1
  Y/1 -> Mux5/1
  Z/1 -> Mux1/1
  Mux1/1 -> Driver Actuator Z/1
  connections:
  Linear Driver Y/RConn1 -- target/RConn2
  Linear Driver X/RConn1 -- target/RConn3
  Weld/RConn1 -- origin/LConn1
  Driver Actuator X/RConn1 -- Linear Driver X/LConn2
  Driver Actuator Y/RConn1 -- Linear Driver Y/LConn2
  Machine Environment/RConn1 -- Ground/LConn1
  Ground/RConn1 -- Weld/LConn1
  Driver Actuator Z/RConn1 -- Linear Driver Z/LConn2
  Linear Driver Z/RConn1 -- target/RConn1
  Custom Joint/RConn1 -- target/LConn1
  Custom Joint/LConn1 -- origin/LConn2
  origin/RConn2 -- Linear Driver Y/LConn1
  origin/RConn3 -- Linear Driver Z/LConn1
  Linear Driver X/LConn1 -- origin/RConn1

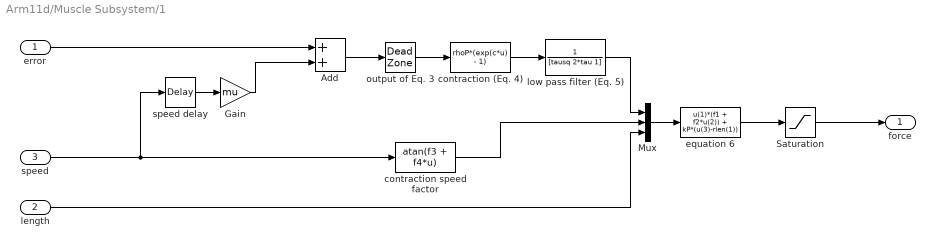
== system Arm11d/Muscle Subsystem/1 ==
  error : Inport
  length : Inport  Port=2
  speed : Inport  Port=3
  Add : Sum
  Gain : Gain  Gain=mu
  Mux : Mux  Inputs=3
  Saturation : Saturate  UpperLimit=1000  LowerLimit=0  ZeroCross=off
  contraction (Eq. 4) : Fcn  Expr=rhoP*(exp(c*u) - 1)
  contraction speed factor : MATLABFcn  MATLABFcn=atan(f3 + f4*u)
  equation 6 : Fcn  Expr=u(1)*(f1 + f2*u(2)) + kP*(u(3)-rlen(1))
  low pass filter (Eq. 5) : TransferFcn  Denominator=[tausq 2*tau 1]
  output of Eq. 3 : DeadZone  LowerValue=-inf  UpperValue=0  ZeroCross=off  SaturateOnIntegerOverflow=on
  speed delay : TransportDelay  DelayTime=d  InitialOutput=.01  BufferSize=20000  TransDelayFeedthrough=on  PadeOrder=1
  force : Outport
  wires:
  Saturation/1 -> force/1
  equation 6/1 -> Saturation/1
  contraction speed factor/1 -> Mux/2
  speed/1 -> contraction speed factor/1, speed delay/1
  length/1 -> Mux/3
  Mux/1 -> equation 6/1
  low pass filter (Eq. 5)/1 -> Mux/1
  contraction (Eq. 4)/1 -> low pass filter (Eq. 5)/1
  output of Eq. 3/1 -> contraction (Eq. 4)/1
  Add/1 -> output of Eq. 3/1
  error/1 -> Add/1
  Gain/1 -> Add/2
  speed delay/1 -> Gain/1

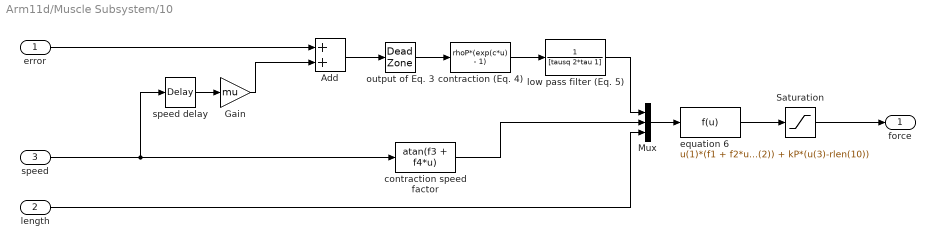
== system Arm11d/Muscle Subsystem/10 ==
  error : Inport
  length : Inport  Port=2
  speed : Inport  Port=3
  Add : Sum
  Gain : Gain  Gain=mu
  Mux : Mux  Inputs=3
  Saturation : Saturate  UpperLimit=1000  LowerLimit=0  ZeroCross=off
  contraction (Eq. 4) : Fcn  Expr=rhoP*(exp(c*u) - 1)
  contraction speed factor : MATLABFcn  MATLABFcn=atan(f3 + f4*u)
  equation 6 : Fcn  Expr=u(1)*(f1 + f2*u(2)) + kP*(u(3)-rlen(10))
  low pass filter (Eq. 5) : TransferFcn  Denominator=[tausq 2*tau 1]
  output of Eq. 3 : DeadZone  LowerValue=-inf  UpperValue=0  ZeroCross=off  SaturateOnIntegerOverflow=on
  speed delay : TransportDelay  DelayTime=d  InitialOutput=.01  BufferSize=20000  TransDelayFeedthrough=on  PadeOrder=1
  force : Outport
  wires:
  Saturation/1 -> force/1
  equation 6/1 -> Saturation/1
  contraction speed factor/1 -> Mux/2
  speed/1 -> contraction speed factor/1, speed delay/1
  length/1 -> Mux/3
  Mux/1 -> equation 6/1
  low pass filter (Eq. 5)/1 -> Mux/1
  contraction (Eq. 4)/1 -> low pass filter (Eq. 5)/1
  output of Eq. 3/1 -> contraction (Eq. 4)/1
  Add/1 -> output of Eq. 3/1
  error/1 -> Add/1
  Gain/1 -> Add/2
  speed delay/1 -> Gain/1

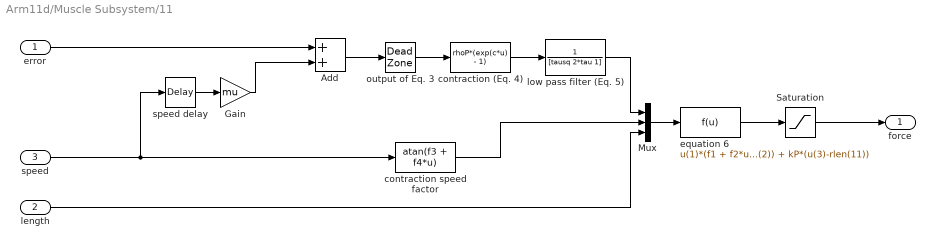
== system Arm11d/Muscle Subsystem/11 ==
  error : Inport
  length : Inport  Port=2
  speed : Inport  Port=3
  Add : Sum
  Gain : Gain  Gain=mu
  Mux : Mux  Inputs=3
  Saturation : Saturate  UpperLimit=1000  LowerLimit=0  ZeroCross=off
  contraction (Eq. 4) : Fcn  Expr=rhoP*(exp(c*u) - 1)
  contraction speed factor : MATLABFcn  MATLABFcn=atan(f3 + f4*u)
  equation 6 : Fcn  Expr=u(1)*(f1 + f2*u(2)) + kP*(u(3)-rlen(11))
  low pass filter (Eq. 5) : TransferFcn  Denominator=[tausq 2*tau 1]
  output of Eq. 3 : DeadZone  LowerValue=-inf  UpperValue=0  ZeroCross=off  SaturateOnIntegerOverflow=on
  speed delay : TransportDelay  DelayTime=d  InitialOutput=.01  BufferSize=20000  TransDelayFeedthrough=on  PadeOrder=1
  force : Outport
  wires:
  Saturation/1 -> force/1
  equation 6/1 -> Saturation/1
  contraction speed factor/1 -> Mux/2
  speed/1 -> contraction speed factor/1, speed delay/1
  length/1 -> Mux/3
  Mux/1 -> equation 6/1
  low pass filter (Eq. 5)/1 -> Mux/1
  contraction (Eq. 4)/1 -> low pass filter (Eq. 5)/1
  output of Eq. 3/1 -> contraction (Eq. 4)/1
  Add/1 -> output of Eq. 3/1
  error/1 -> Add/1
  Gain/1 -> Add/2
  speed delay/1 -> Gain/1

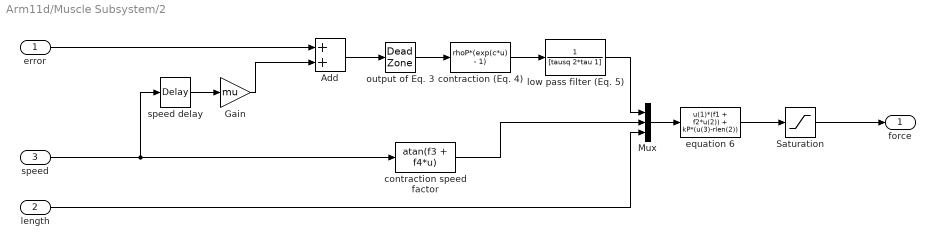
== system Arm11d/Muscle Subsystem/2 ==
  error : Inport
  length : Inport  Port=2
  speed : Inport  Port=3
  Add : Sum
  Gain : Gain  Gain=mu
  Mux : Mux  Inputs=3
  Saturation : Saturate  UpperLimit=1000  LowerLimit=0  ZeroCross=off
  contraction (Eq. 4) : Fcn  Expr=rhoP*(exp(c*u) - 1)
  contraction speed factor : MATLABFcn  MATLABFcn=atan(f3 + f4*u)
  equation 6 : Fcn  Expr=u(1)*(f1 + f2*u(2)) + kP*(u(3)-rlen(2))
  low pass filter (Eq. 5) : TransferFcn  Denominator=[tausq 2*tau 1]
  output of Eq. 3 : DeadZone  LowerValue=-inf  UpperValue=0  ZeroCross=off  SaturateOnIntegerOverflow=on
  speed delay : TransportDelay  DelayTime=d  InitialOutput=.01  BufferSize=20000  TransDelayFeedthrough=on  PadeOrder=1
  force : Outport
  wires:
  Saturation/1 -> force/1
  equation 6/1 -> Saturation/1
  contraction speed factor/1 -> Mux/2
  speed/1 -> contraction speed factor/1, speed delay/1
  length/1 -> Mux/3
  Mux/1 -> equation 6/1
  low pass filter (Eq. 5)/1 -> Mux/1
  contraction (Eq. 4)/1 -> low pass filter (Eq. 5)/1
  output of Eq. 3/1 -> contraction (Eq. 4)/1
  Add/1 -> output of Eq. 3/1
  error/1 -> Add/1
  Gain/1 -> Add/2
  speed delay/1 -> Gain/1

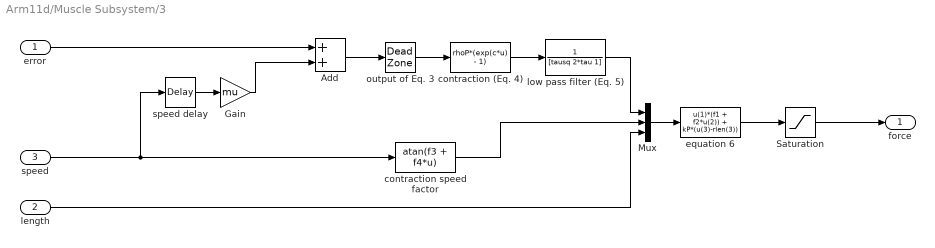
== system Arm11d/Muscle Subsystem/3 ==
  error : Inport
  length : Inport  Port=2
  speed : Inport  Port=3
  Add : Sum
  Gain : Gain  Gain=mu
  Mux : Mux  Inputs=3
  Saturation : Saturate  UpperLimit=1000  LowerLimit=0  ZeroCross=off
  contraction (Eq. 4) : Fcn  Expr=rhoP*(exp(c*u) - 1)
  contraction speed factor : MATLABFcn  MATLABFcn=atan(f3 + f4*u)
  equation 6 : Fcn  Expr=u(1)*(f1 + f2*u(2)) + kP*(u(3)-rlen(3))
  low pass filter (Eq. 5) : TransferFcn  Denominator=[tausq 2*tau 1]
  output of Eq. 3 : DeadZone  LowerValue=-inf  UpperValue=0  ZeroCross=off  SaturateOnIntegerOverflow=on
  speed delay : TransportDelay  DelayTime=d  InitialOutput=.01  BufferSize=20000  TransDelayFeedthrough=on  PadeOrder=1
  force : Outport
  wires:
  Saturation/1 -> force/1
  equation 6/1 -> Saturation/1
  contraction speed factor/1 -> Mux/2
  speed/1 -> contraction speed factor/1, speed delay/1
  length/1 -> Mux/3
  Mux/1 -> equation 6/1
  low pass filter (Eq. 5)/1 -> Mux/1
  contraction (Eq. 4)/1 -> low pass filter (Eq. 5)/1
  output of Eq. 3/1 -> contraction (Eq. 4)/1
  Add/1 -> output of Eq. 3/1
  error/1 -> Add/1
  Gain/1 -> Add/2
  speed delay/1 -> Gain/1

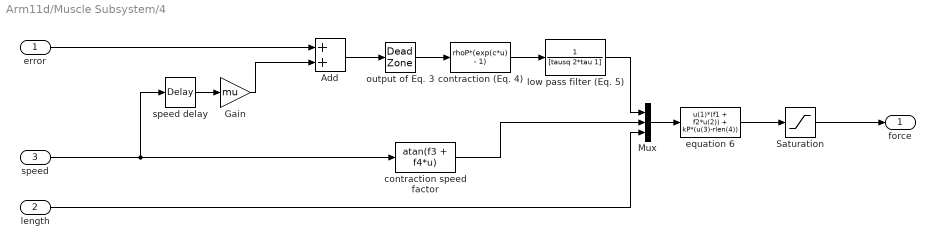
== system Arm11d/Muscle Subsystem/4 ==
  error : Inport
  length : Inport  Port=2
  speed : Inport  Port=3
  Add : Sum
  Gain : Gain  Gain=mu
  Mux : Mux  Inputs=3
  Saturation : Saturate  UpperLimit=1000  LowerLimit=0  ZeroCross=off
  contraction (Eq. 4) : Fcn  Expr=rhoP*(exp(c*u) - 1)
  contraction speed factor : MATLABFcn  MATLABFcn=atan(f3 + f4*u)
  equation 6 : Fcn  Expr=u(1)*(f1 + f2*u(2)) + kP*(u(3)-rlen(4))
  low pass filter (Eq. 5) : TransferFcn  Denominator=[tausq 2*tau 1]
  output of Eq. 3 : DeadZone  LowerValue=-inf  UpperValue=0  ZeroCross=off  SaturateOnIntegerOverflow=on
  speed delay : TransportDelay  DelayTime=d  InitialOutput=.01  BufferSize=20000  TransDelayFeedthrough=on  PadeOrder=1
  force : Outport
  wires:
  Saturation/1 -> force/1
  equation 6/1 -> Saturation/1
  contraction speed factor/1 -> Mux/2
  speed/1 -> contraction speed factor/1, speed delay/1
  length/1 -> Mux/3
  Mux/1 -> equation 6/1
  low pass filter (Eq. 5)/1 -> Mux/1
  contraction (Eq. 4)/1 -> low pass filter (Eq. 5)/1
  output of Eq. 3/1 -> contraction (Eq. 4)/1
  Add/1 -> output of Eq. 3/1
  error/1 -> Add/1
  Gain/1 -> Add/2
  speed delay/1 -> Gain/1

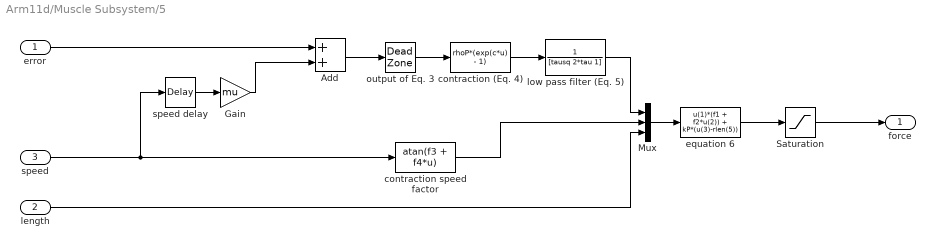
== system Arm11d/Muscle Subsystem/5 ==
  error : Inport
  length : Inport  Port=2
  speed : Inport  Port=3
  Add : Sum
  Gain : Gain  Gain=mu
  Mux : Mux  Inputs=3
  Saturation : Saturate  UpperLimit=1000  LowerLimit=0  ZeroCross=off
  contraction (Eq. 4) : Fcn  Expr=rhoP*(exp(c*u) - 1)
  contraction speed factor : MATLABFcn  MATLABFcn=atan(f3 + f4*u)
  equation 6 : Fcn  Expr=u(1)*(f1 + f2*u(2)) + kP*(u(3)-rlen(5))
  low pass filter (Eq. 5) : TransferFcn  Denominator=[tausq 2*tau 1]
  output of Eq. 3 : DeadZone  LowerValue=-inf  UpperValue=0  ZeroCross=off  SaturateOnIntegerOverflow=on
  speed delay : TransportDelay  DelayTime=d  InitialOutput=.01  BufferSize=20000  TransDelayFeedthrough=on  PadeOrder=1
  force : Outport
  wires:
  Saturation/1 -> force/1
  equation 6/1 -> Saturation/1
  contraction speed factor/1 -> Mux/2
  speed/1 -> contraction speed factor/1, speed delay/1
  length/1 -> Mux/3
  Mux/1 -> equation 6/1
  low pass filter (Eq. 5)/1 -> Mux/1
  contraction (Eq. 4)/1 -> low pass filter (Eq. 5)/1
  output of Eq. 3/1 -> contraction (Eq. 4)/1
  Add/1 -> output of Eq. 3/1
  error/1 -> Add/1
  Gain/1 -> Add/2
  speed delay/1 -> Gain/1

== system Arm11d/Muscle Subsystem/6 ==
  error : Inport
  length : Inport  Port=2
  speed : Inport  Port=3
  Add : Sum
  Gain : Gain  Gain=mu
  Mux : Mux  Inputs=3
  Saturation : Saturate  UpperLimit=1000  LowerLimit=0  ZeroCross=off
  contraction (Eq. 4) : Fcn  Expr=rhoP*(exp(c*u) - 1)
  contraction speed factor : MATLABFcn  MATLABFcn=atan(f3 + f4*u)
  equation 6 : Fcn  Expr=u(1)*(f1 + f2*u(2)) + kP*(u(3)-rlen(6))
  low pass filter (Eq. 5) : TransferFcn  Denominator=[tausq 2*tau 1]
  output of Eq. 3 : DeadZone  LowerValue=-inf  UpperValue=0  ZeroCross=off  SaturateOnIntegerOverflow=on
  speed delay : TransportDelay  DelayTime=d  InitialOutput=.01  BufferSize=20000  TransDelayFeedthrough=on  PadeOrder=1
  force : Outport
  wires:
  Saturation/1 -> force/1
  equation 6/1 -> Saturation/1
  contraction speed factor/1 -> Mux/2
  speed/1 -> contraction speed factor/1, speed delay/1
  length/1 -> Mux/3
  Mux/1 -> equation 6/1
  low pass filter (Eq. 5)/1 -> Mux/1
  contraction (Eq. 4)/1 -> low pass filter (Eq. 5)/1
  output of Eq. 3/1 -> contraction (Eq. 4)/1
  Add/1 -> output of Eq. 3/1
  error/1 -> Add/1
  Gain/1 -> Add/2
  speed delay/1 -> Gain/1

== system Arm11d/Muscle Subsystem/7 ==
  error : Inport
  length : Inport  Port=2
  speed : Inport  Port=3
  Add : Sum
  Gain : Gain  Gain=mu
  Mux : Mux  Inputs=3
  Saturation : Saturate  UpperLimit=1000  LowerLimit=0  ZeroCross=off
  contraction (Eq. 4) : Fcn  Expr=rhoP*(exp(c*u) - 1)
  contraction speed factor : MATLABFcn  MATLABFcn=atan(f3 + f4*u)
  equation 6 : Fcn  Expr=u(1)*(f1 + f2*u(2)) + kP*(u(3)-rlen(7))
  low pass filter (Eq. 5) : TransferFcn  Denominator=[tausq 2*tau 1]
  output of Eq. 3 : DeadZone  LowerValue=-inf  UpperValue=0  ZeroCross=off  SaturateOnIntegerOverflow=on
  speed delay : TransportDelay  DelayTime=d  InitialOutput=.01  BufferSize=20000  TransDelayFeedthrough=on  PadeOrder=1
  force : Outport
  wires:
  Saturation/1 -> force/1
  equation 6/1 -> Saturation/1
  contraction speed factor/1 -> Mux/2
  speed/1 -> contraction speed factor/1, speed delay/1
  length/1 -> Mux/3
  Mux/1 -> equation 6/1
  low pass filter (Eq. 5)/1 -> Mux/1
  contraction (Eq. 4)/1 -> low pass filter (Eq. 5)/1
  output of Eq. 3/1 -> contraction (Eq. 4)/1
  Add/1 -> output of Eq. 3/1
  error/1 -> Add/1
  Gain/1 -> Add/2
  speed delay/1 -> Gain/1

== system Arm11d/Muscle Subsystem/8 ==
  error : Inport
  length : Inport  Port=2
  speed : Inport  Port=3
  Add : Sum
  Gain : Gain  Gain=mu
  Mux : Mux  Inputs=3
  Saturation : Saturate  UpperLimit=1000  LowerLimit=0  ZeroCross=off
  contraction (Eq. 4) : Fcn  Expr=rhoP*(exp(c*u) - 1)
  contraction speed factor : MATLABFcn  MATLABFcn=atan(f3 + f4*u)
  equation 6 : Fcn  Expr=u(1)*(f1 + f2*u(2)) + kP*(u(3)-rlen(8))
  low pass filter (Eq. 5) : TransferFcn  Denominator=[tausq 2*tau 1]
  output of Eq. 3 : DeadZone  LowerValue=-inf  UpperValue=0  ZeroCross=off  SaturateOnIntegerOverflow=on
  speed delay : TransportDelay  DelayTime=d  InitialOutput=.01  BufferSize=20000  TransDelayFeedthrough=on  PadeOrder=1
  force : Outport
  wires:
  Saturation/1 -> force/1
  equation 6/1 -> Saturation/1
  contraction speed factor/1 -> Mux/2
  speed/1 -> contraction speed factor/1, speed delay/1
  length/1 -> Mux/3
  Mux/1 -> equation 6/1
  low pass filter (Eq. 5)/1 -> Mux/1
  contraction (Eq. 4)/1 -> low pass filter (Eq. 5)/1
  output of Eq. 3/1 -> contraction (Eq. 4)/1
  Add/1 -> output of Eq. 3/1
  error/1 -> Add/1
  Gain/1 -> Add/2
  speed delay/1 -> Gain/1

== system Arm11d/Muscle Subsystem/9 ==
  error : Inport
  length : Inport  Port=2
  speed : Inport  Port=3
  Add : Sum
  Gain : Gain  Gain=mu
  Mux : Mux  Inputs=3
  Saturation : Saturate  UpperLimit=1000  LowerLimit=0  ZeroCross=off
  contraction (Eq. 4) : Fcn  Expr=rhoP*(exp(c*u) - 1)
  contraction speed factor : MATLABFcn  MATLABFcn=atan(f3 + f4*u)
  equation 6 : Fcn  Expr=u(1)*(f1 + f2*u(2)) + kP*(u(3)-rlen(9))
  low pass filter (Eq. 5) : TransferFcn  Denominator=[tausq 2*tau 1]
  output of Eq. 3 : DeadZone  LowerValue=-inf  UpperValue=0  ZeroCross=off  SaturateOnIntegerOverflow=on
  speed delay : TransportDelay  DelayTime=d  InitialOutput=.01  BufferSize=20000  TransDelayFeedthrough=on  PadeOrder=1
  force : Outport
  wires:
  Saturation/1 -> force/1
  equation 6/1 -> Saturation/1
  contraction speed factor/1 -> Mux/2
  speed/1 -> contraction speed factor/1, speed delay/1
  length/1 -> Mux/3
  Mux/1 -> equation 6/1
  low pass filter (Eq. 5)/1 -> Mux/1
  contraction (Eq. 4)/1 -> low pass filter (Eq. 5)/1
  output of Eq. 3/1 -> contraction (Eq. 4)/1
  Add/1 -> output of Eq. 3/1
  error/1 -> Add/1
  Gain/1 -> Add/2
  speed delay/1 -> Gain/1
